simulink model "Single_Phase_Differential_Buck_Inverter"  (R2022b)
settings: Solver=VariableStepAuto  StartTime=0.0  StopTime=10.0  RelTol=1e-3
libraries: spsSeriesRLCBranchLib x5, spsMosfetLib x4, spsVoltageMeasurementLib x3, spsTriangleGeneratorLib x2, spsDCVoltageSourceLib x1, spspowerguiLib x1
settings Model: Creator=nishi  LastModifiedBy=nishi

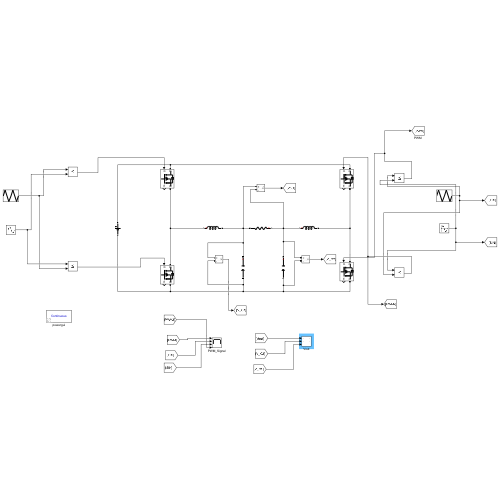
[thumbnail: Simulink's stored preview of the top-level diagram]
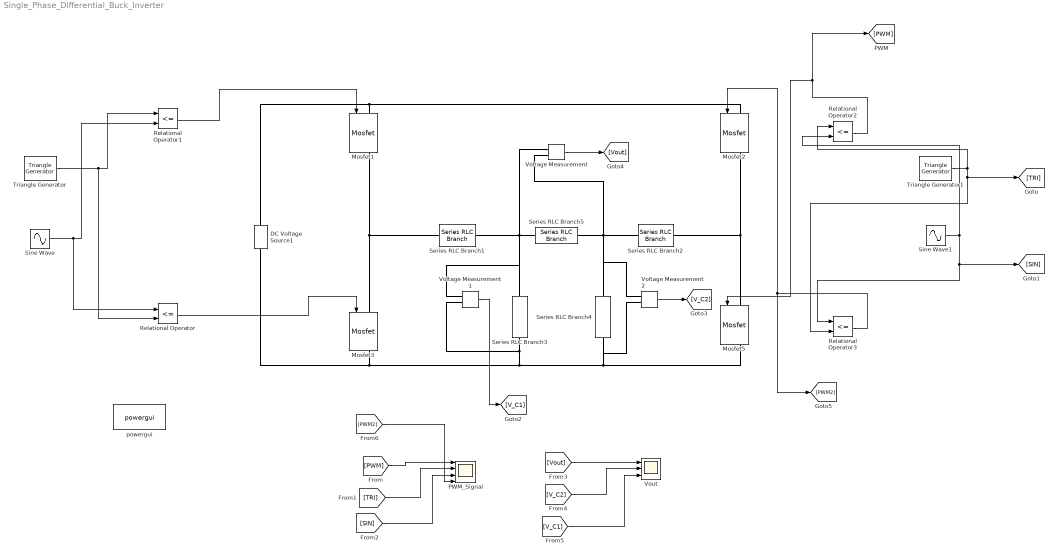
== system Single_Phase_Differential_Buck_Inverter ==
  DC Voltage Source1 : spsDCVoltageSourceLib/DC Voltage Source  Amplitude=100  Measurements=None
  Mosfet{1..3,5} (4 alike) : spsMosfetLib/Mosfet  Ron=1e-7  Lon=0  Rd=1e-10  Vfd=0  IC=0  Rs=inf  Cs=0  Measurements=on
  PWM_Signal : Scope  NumInputPorts=4
  Relational Operator{,1..3} (4 alike) : RelationalOperator  Operator=<=  OutDataTypeStr=boolean  RndMeth=Simplest  InputSameDT=off
  Series RLC Branch1 : spsSeriesRLCBranchLib/Series RLC Branch  LConnTagsString=__new0  RConnTagsString=__new0  BranchType=L  Resistance=0.000001  Inductance=0.004  SetiL0=off  InitialCurrent=0  Capacitance=1e-6  Setx0=off  InitialVoltage=0  Measurements=None
  Series RLC Branch2 : spsSeriesRLCBranchLib/Series RLC Branch  LConnTagsString=__new0  RConnTagsString=__new0  BranchType=L  Resistance=0.000001  Inductance=0.004  SetiL0=off  InitialCurrent=0  Capacitance=1e-6  Setx0=off  InitialVoltage=0  Measurements=None
  Series RLC Branch3 : spsSeriesRLCBranchLib/Series RLC Branch  LConnTagsString=__new0  RConnTagsString=__new0  BranchType=C  Resistance=6  Inductance=1e-3  SetiL0=off  InitialCurrent=0  Capacitance=5e-6  Setx0=off  InitialVoltage=800  Measurements=None
  Series RLC Branch4 : spsSeriesRLCBranchLib/Series RLC Branch  LConnTagsString=__new0  RConnTagsString=__new0  BranchType=C  Resistance=6  Inductance=1e-3  SetiL0=off  InitialCurrent=0  Capacitance=5e-6  Setx0=off  InitialVoltage=800  Measurements=None
  Series RLC Branch5 : spsSeriesRLCBranchLib/Series RLC Branch  LConnTagsString=__new0  RConnTagsString=__new0  BranchType=R  Resistance=100  Inductance=1e-3  SetiL0=off  InitialCurrent=0  Capacitance=1000e-6  Setx0=on  InitialVoltage=800  Measurements=None
  Sine Wave : Sin  Frequency=314.16  SampleTime=0
  Sine Wave1 : Sin  Frequency=314.16  SampleTime=0
  Triangle Generator : spsTriangleGeneratorLib/Triangle Generator  Freq=20000  Phase=90  Ts=0
  Triangle Generator1 : spsTriangleGeneratorLib/Triangle Generator  Freq=20000  Phase=90  Ts=0
  Voltage Measurement : spsVoltageMeasurementLib/Voltage Measurement  PhasorSimulation=off  OutputType=Complex  PSBequivalent=0
  Voltage Measurement1 : spsVoltageMeasurementLib/Voltage Measurement  PhasorSimulation=off  OutputType=Complex  PSBequivalent=0
  Voltage Measurement2 : spsVoltageMeasurementLib/Voltage Measurement  PhasorSimulation=off  OutputType=Complex  PSBequivalent=0
  Vout : Scope  NumInputPorts=3
  powergui : spspowerguiLib/powergui  Priority=1  SimulationMode=Continuous  SampleTime=50e-6  frequency=60  Iterations=50  frequencyindice=0  Pbase=100e6  ErrMax=1e-4  UnitsV=kV  UnitsW=MW  buscounter=0  FunctionMessages=off  echomessages=off  EnableUseOfTLC=off  CurrentSourceSwitches=off  DisableSnubberDevices=off  DisableRonSwitches=off  DisableVfSwitches=off  DisplayEquations=off  AutomaticDiscreteSolvers=off  SolverType=Tustin/Backward Euler (TBE)  Interpol=off  ExternalGateDelay=off  methode=off  Ts=100  x0status=blocks  SPID=on  SwTol=0  HookPort=off  NonlinearTolerance=1e-4  nMaxIteration=100  ContinueOnMaxIteration=off  RestoreLinks=warning  ResistiveCurrentMeasurement=off  Frange=[0:2:500]  Ylog=off  Xlog=on  ShowGrid=off  save=off  variable=ZData  structure=0  ZoomFFT=off  StartTime=0.0  cycles=1  DisplayStyle=1  fundamental=60  FreqAxis=off  MaxFrequency=1000  frequencyindicesteady=1  RmsSteady=1  display=off
  wires:
  Triangle Generator/1 -> Relational Operator/2, Relational Operator1/1
  Sine Wave/1 -> Relational Operator/1, Relational Operator1/2
  Relational Operator1/1 -> Mosfet1/1
  Relational Operator/1 -> Mosfet3/1
  Triangle Generator1/1 -> [TRI], Relational Operator3/2, Relational Operator2/1
  Sine Wave1/1 -> [SIN], Relational Operator3/1, Relational Operator2/2
  Relational Operator2/1 -> Mosfet5/1, [PWM]
  [PWM] -> PWM_Signal/1
  [TRI] -> PWM_Signal/2
  [SIN] -> PWM_Signal/3
  Voltage Measurement/1 -> [Vout]
  [Vout] -> Vout/1
  Voltage Measurement2/1 -> [V_C2]
  Voltage Measurement1/1 -> [V_C1]
  [V_C2] -> Vout/2
  [V_C1] -> Vout/3
  [PWM2] -> PWM_Signal/4
  Relational Operator3/1 -> [PWM2], Mosfet2/1
  connections:
  Mosfet1/RConn1 -- Series RLC Branch1/LConn1 -- Mosfet3/LConn1
  Mosfet3/RConn1 -- Voltage Measurement2/LConn2 -- Series RLC Branch4/RConn1 -- Mosfet5/RConn1 -- Voltage Measurement1/LConn2 -- Series RLC Branch3/RConn1 -- DC Voltage Source1/LConn1
  Mosfet5/LConn1 -- Series RLC Branch2/RConn1 -- Mosfet2/RConn1
  Mosfet1/LConn1 -- Mosfet2/LConn1 -- DC Voltage Source1/RConn1
  Series RLC Branch1/RConn1 -- Voltage Measurement1/LConn1 -- Series RLC Branch3/LConn1 -- Voltage Measurement/LConn1 -- Series RLC Branch5/RConn1
  Series RLC Branch5/LConn1 -- Voltage Measurement2/LConn1 -- Series RLC Branch4/LConn1 -- Voltage Measurement/LConn2 -- Series RLC Branch2/LConn1
